simulink model "saturated_roll_system"  (R2019b)
settings: Solver=VariableStepAuto  StartTime=0.0  StopTime=10.0  RelTol=1e-3
undefined symbols (not defined in the file or in its folder): G_phi_samples
libraries: cstblocks x5
settings Model: Creator=amirhossein  LastModifiedBy=amirhossein

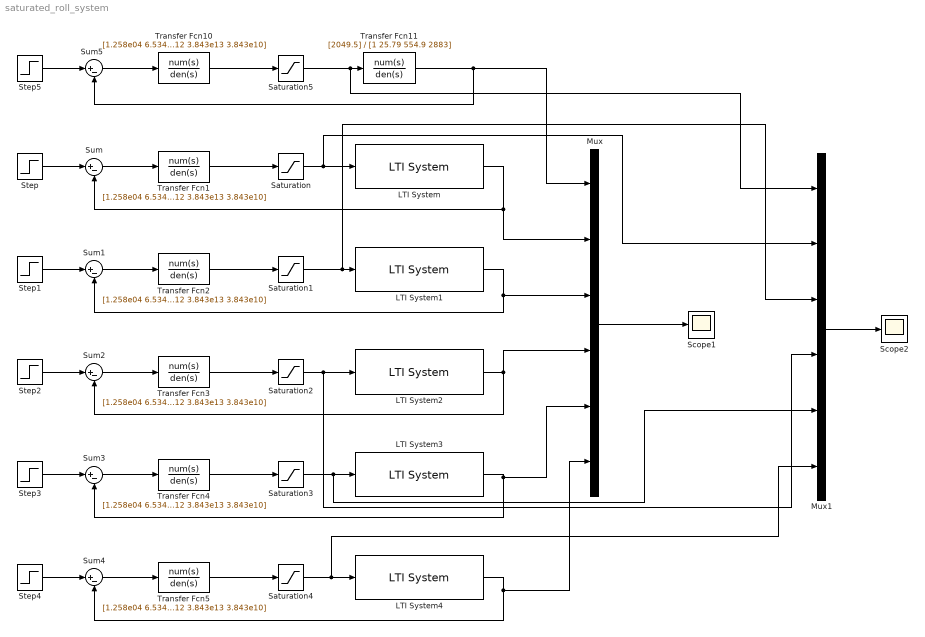
== system saturated_roll_system ==
  LTI System : cstblocks/LTI System  sys=G_phi_samples(: , : , 1)  IC=[]
  LTI System1 : cstblocks/LTI System  sys=G_phi_samples(: , : , 2)  IC=[]
  LTI System2 : cstblocks/LTI System  sys=G_phi_samples(: , : , 3)  IC=[]
  LTI System3 : cstblocks/LTI System  sys=G_phi_samples(: , : , 4)  IC=[]
  LTI System4 : cstblocks/LTI System  sys=G_phi_samples(: , : , 5)  IC=[]
  Mux : Mux  Inputs=6
  Mux1 : Mux  Inputs=6
  Saturation{,1..5} (6 alike) : Saturate  UpperLimit=20  LowerLimit=-20
  Scope1 : Scope
  Scope2 : Scope
  Step{,1..5} (6 alike) : Step  SampleTime=0
  Sum{,1..5} (6 alike) : Sum  Inputs=|+-
  Transfer Fcn{1..5,10} (6 alike) : TransferFcn  Numerator=[1.258e04 6.534e06 6.665e08 3.016e10 7.851e11 1.256e13 1.142e14 3.868e14]  Denominator=[1 2032 1.172e06 1.496e08 9.86e09 3.484e11 5.991e12 3.843e13 3.843e10]
  Transfer Fcn11 : TransferFcn  Numerator=[2049.5]  Denominator=[1 25.79 554.9 2883]
  wires:
  Transfer Fcn1/1 -> Saturation/1
  LTI System3/1 -> Mux/5, Sum3/2
  Saturation5/1 -> Mux1/1, Transfer Fcn11/1
  Saturation2/1 -> Mux1/4, LTI System2/1
  LTI System1/1 -> Mux/3, Sum1/2
  Sum2/1 -> Transfer Fcn3/1
  Transfer Fcn10/1 -> Saturation5/1
  Step3/1 -> Sum3/1
  Saturation/1 -> Mux1/2, LTI System/1
  Sum5/1 -> Transfer Fcn10/1
  Step/1 -> Sum/1
  Sum/1 -> Transfer Fcn1/1
  Transfer Fcn4/1 -> Saturation3/1
  Sum4/1 -> Transfer Fcn5/1
  Step5/1 -> Sum5/1
  LTI System/1 -> Mux/2, Sum/2
  Step1/1 -> Sum1/1
  Transfer Fcn2/1 -> Saturation1/1
  Mux/1 -> Scope1/1
  LTI System2/1 -> Mux/4, Sum2/2
  Transfer Fcn11/1 -> Sum5/2, Mux/1
  Sum1/1 -> Transfer Fcn2/1
  Step2/1 -> Sum2/1
  Transfer Fcn5/1 -> Saturation4/1
  Saturation3/1 -> Mux1/5, LTI System3/1
  Saturation1/1 -> Mux1/3, LTI System1/1
  LTI System4/1 -> Mux/6, Sum4/2
  Sum3/1 -> Transfer Fcn4/1
  Transfer Fcn3/1 -> Saturation2/1
  Step4/1 -> Sum4/1
  Saturation4/1 -> Mux1/6, LTI System4/1
  Mux1/1 -> Scope2/1
